simulink model "darko_control_lineaire_wind_test"  (R2021b)
settings: Solver=VariableStepAuto  StartTime=0.0  StopTime=50  RelTol=1e-3
values from neighbouring files (symbols this model uses):
  C = [C(1:7,:);C(9:12,:)]    [main_linearisation_wi.m]
  drone = generateDarko()    [equilibre.m]    (also in generateDarko.m = struct('MASS',               0.400,                      'IN; main_linearisation_wi.m)
  initial_state = [p_initial; v_initial; q_initial; omega_initial]    [main_linearisation_wi.m]
  K_complet = [K(:,1:6), zeros(4,1), K(:,7:12)]    [main_linearisation_wi.m]
  solution = fmincon(fun,x0,[],[],[],[],lb,ub, [], options)    [main_linearisation_wi.m]
  u_eq = drone.G*drone.MASS/(2*drone.Fb(1,1)) * [1;1;0;0]    [main_linearisation_wi.m]
  x_eq = [[0; 0; 0]; [0; 0; 0]; [1/sqrt(2); 0; 1/sqrt(2);0]; [0; 0; 0]]    [main_linearisation_wi.m]
  x_eq_ = [[0; 0; 0]; [0; 0; 0]; [0; 0]; [0; 0; 0]]    [main_linearisation_wi.m]
libraries: simulink_extras x11, aerolibanim x1, sharedtransform x1
settings Model: Creator=florian  LastModifiedBy=florian
settings SolverCC: AlgebraicLoopSolver=TrustRegion
settings DebuggingCC: SFMachineParentedDataDiag=warning

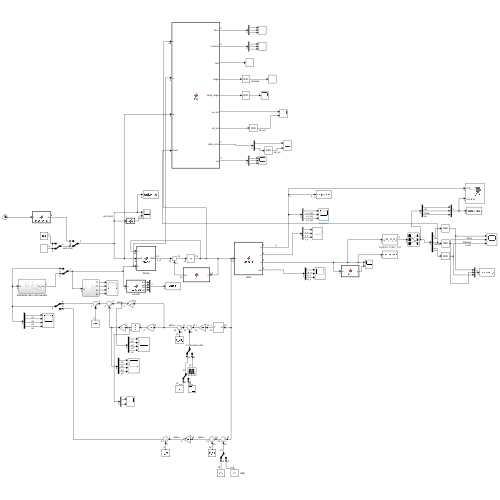
[thumbnail: Simulink's stored preview of the top-level diagram]
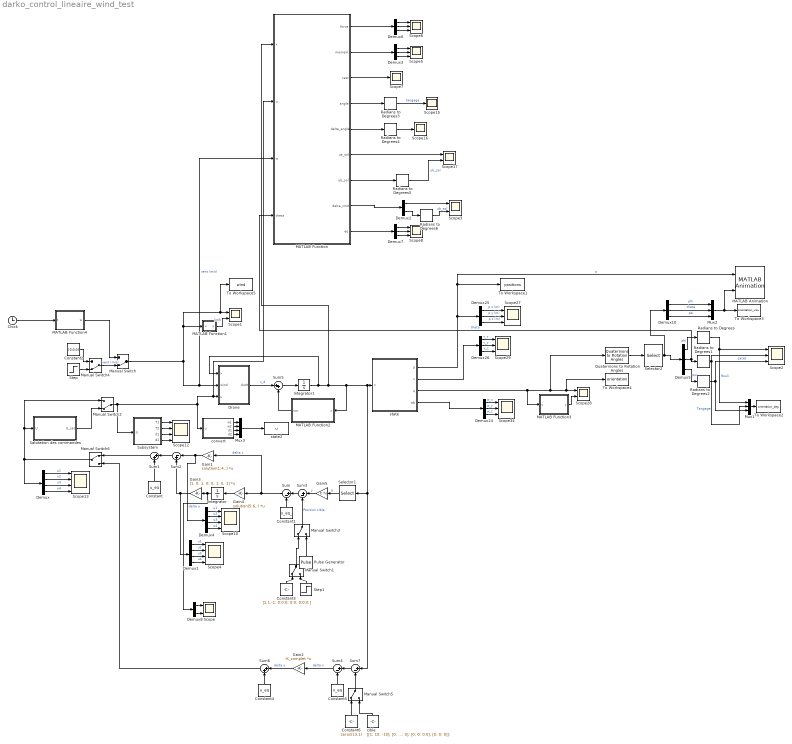
== system darko_control_lineaire_wind_test ==
  Clock : Clock
  Constant : Constant  Value=u_eq
  Constant1 : Constant  Value=x_eq_
  Constant2 : Constant  Value=[0;0;0]
  Constant3 : Constant  Value=[1;1;-1; 0;0;0; 0;0; 0;0;0;]
  Constant4 : Constant  Value=u_eq
  Constant5 : Constant  Value=x_eq
  Constant6 : Constant  Value=zeros(13,1)
  Demux : Demux
  Demux1 : Demux
  Demux{3,5..7,10,24..26} (8 alike) : Demux  Outputs=3
  Demux2 : Demux  Outputs=2
  Demux4 : Demux
  Demux8 : Demux  Outputs=2
  Drone : MATLAB Function  TreatAsAtomicUnit=on
  Gain1 : Gain  Gain=solution(1:4,:)  Multiplication=Matrix(K*u) (u vector)
  Gain2 : Gain  Gain=-K_complet  Multiplication=Matrix(K*u) (u vector)
  Gain3 : Gain  Gain=[1, 0; 1, 0; 0, 1; 0, 1]  Multiplication=Matrix(K*u) (u vector)
  Gain4 : Gain  Gain=solution(5:6,:)  Multiplication=Matrix(K*u) (u vector)
  Gain5 : Gain  Gain=C  Multiplication=Matrix(K*u) (u vector)
  Integrator : Integrator  InitialCondition=zeros(1,2)
  Integrator1 : Integrator  InitialCondition=initial_state
  MATLAB Animation : aerolibanim/MATLAB Animation  Tag=Matlab Animation 6 DOF  Vehicles=1  Geometries='astredwedge.mat'  BoundingBoxCoordinates=[-50,50,-50,50,-50,50]  CameraOffset=[0,-50,0]  CameraViewAngle=10  SampleTime=0.08  FigurePosition=[635,-23,492,413]
      settings: SourceProductBaseCode=AE
  MATLAB Function : MATLAB Function  TreatAsAtomicUnit=on
  MATLAB Function1 : MATLAB Function  TreatAsAtomicUnit=on
  MATLAB Function2 : MATLAB Function  TreatAsAtomicUnit=on
  MATLAB Function3 : MATLAB Function  TreatAsAtomicUnit=on
  MATLAB Function4 : MATLAB Function  TreatAsAtomicUnit=on
  Manual Switch : ManualSwitch  CurrentSetting=0
  Manual Switch{1,3,5..6} (4 alike) : ManualSwitch
  Manual Switch2 : ManualSwitch  CurrentSetting=0
  Manual Switch4 : ManualSwitch  CurrentSetting=0
  Mux1 : Mux  Inputs=3
  Mux2 : Mux  Inputs=3
  Mux3 : Mux
  Pulse Generator : DiscretePulseGenerator  PulseType=Time based  Amplitude=[0;0;-5; 0;0;0; 0;0; 0;0;0]  Period=5  PulseWidth=50
  Quaternions to Rotation Angles : sharedtransform/Quaternions to Rotation Angles  rotationOrder=ZXY  aMode=aMode
      settings: SourceProductBaseCode=AE,PW,DR,MT,UV,VE
  Radians to Degrees{,1..6} (7 alike) : simulink_extras/Transformations/Radians to Degrees
  Satutation des commandes : Subsystem
  Scope{,1,3,17,28} (5 alike) : Scope  NumInputPorts=2
  Scope{4,10,12..13} (4 alike) : Scope  NumInputPorts=4
  Scope15 : Scope
  Scope16 : Scope
  Scope{2,5..6,8,27,29,34} (7 alike) : Scope  NumInputPorts=3
  Scope7 : Scope
  Selector1 : Selector  InputPortWidth=13  IndexOptions=Index vector (dialog)  Indices=[1:6 8:13]  OutputSizes=1
  Selector2 : Selector  InputPortWidth=3  IndexOptions=Index vector (dialog)  Indices=[2 3 1]  OutputSizes=1
  Step : Step  Time=20  Before=[0;0;0]  After=[-4;0;0]  SampleTime=0
  Step1 : Step  Time=35  Before=zeros(11,1)  After=[-0.1;0;0; 0;0;0; 0;0; 0;0;0]  SampleTime=0
  Subsystem : Subsystem
  Sum{,3..4,7} (4 alike) : Sum  Inputs=|+-
  Sum1 : Sum  Inputs=|++
  Sum2 : Sum  Inputs=|-+
  Sum5 : Sum  Inputs=|++
  Sum6 : Sum  Inputs=|++
  To Workspace1 : ToWorkspace  VariableName=positions  SampleTime=-1
  To Workspace2 : ToWorkspace  VariableName=orientation_deg  SampleTime=-1
  To Workspace3 : ToWorkspace  VariableName=orientation_visu  SampleTime=-1
  To Workspace4 : ToWorkspace  VariableName=orientation  SampleTime=-1
  To Workspace5 : ToWorkspace  VariableName=wind  SampleTime=-1
  cible : Constant  Value=[[1; 10; -10]; [0; 0; 0]; [0; 0; 0;0]; [0; 0; 0]];
  convert : MATLAB Function  TreatAsAtomicUnit=on
  state : MATLAB Function  TreatAsAtomicUnit=on
  state2 : ToWorkspace  VariableName=u  SampleTime=-1
  wires:
  Sum5/1 -> Integrator1/1
  MATLAB Function2/1(cor) -> Sum5/2
  Drone/1(dxdt) -> Sum5/1  "x_d"
  Integrator1/1 -> Drone/1(x), MATLAB Function/1(x), Sum7/1, Selector1/1, state/1(x), MATLAB Function2/1(x)
  Demux25/3 -> Scope27/3  "p z (m)"
  Demux26/2 -> Scope29/2  "v_y"
  Demux24/1 -> Scope34/1  "w_x"
  MATLAB Function3/1(y) -> Scope28/2
  Demux25/1 -> Scope27/1  "p x (m)"
  state/4(wb) -> Demux24/1
  Demux24/2 -> Scope34/2  "w_y"
  Demux24/3 -> Scope34/3  "w_z"
  state/2(v) -> Demux26/1
  Demux25/2 -> Scope27/2  "p y (m)"
  Demux26/3 -> Scope29/3  "v_z"
  Demux26/1 -> Scope29/1  "v_x"
  Constant/1 -> Sum1/2
  Constant1/1 -> Sum/2
  Demux5/2 -> MATLAB Function/4(theta), Radians to Degrees1/1  "theta"
  Demux5/1 -> Radians to Degrees/1  "phi"
  Demux5/3 -> Radians to Degrees2/1  "psi"
  Demux/3 -> Scope13/3  "u3"
  Manual Switch6/1 -> Demux/1, Satutation des commandes/1(U), Manual Switch2/1
  Demux/2 -> Scope13/2  "u2"
  Manual Switch2/1 -> Subsystem/1(U), convert/1(u), MATLAB Function/2(u), Drone/3(u)
  Demux/1 -> Scope13/1  "u1"
  Demux/4 -> Scope13/4  "u4"
  Mux1/1 -> To Workspace2/1
  state/3(q) -> Quaternions to Rotation Angles/1, Scope28/1, To Workspace4/1, MATLAB Function3/1(u)
  Satutation des commandes/1(U_sat) -> Manual Switch2/2
  Demux10/2 -> Mux2/2  "theta"
  Selector2/1 -> Demux10/1, Demux5/1
  Demux10/1 -> Mux2/1  "phi"
  Demux10/3 -> Mux2/3  "psi"
  state/1(p) -> Demux25/1, MATLAB Animation/1, To Workspace1/1  "p"
  Mux2/1 -> To Workspace3/1, MATLAB Animation/2
  Manual Switch/1 -> MATLAB Function/3(w), Drone/2(wind), To Workspace5/1, Scope1/1, MATLAB Function1/1(u)  "vent (m/s)"
  Radians to Degrees1/1 -> Mux1/2, Scope2/2  "Tangage"
  Radians to Degrees/1 -> Scope2/1, Mux1/1  "Rouli"
  Radians to Degrees2/1 -> Scope2/3, Mux1/3  "Lacet"
  Integrator/1 -> Demux8/1, Gain3/1
  Sum/1 -> Gain4/1, Gain1/1  "delta x"
  Gain4/1 -> Integrator/1
  Sum2/1 -> Sum1/1
  Gain1/1 -> Demux4/1, Sum2/1  "delta u"
  Demux1/2 -> Scope4/2  "u2"
  Demux1/3 -> Scope4/3  "u3"
  Demux1/4 -> Scope4/4  "u4"
  Demux1/1 -> Scope4/1  "u1"
  Gain5/1 -> Sum3/1  "y"
  Sum3/1 -> Sum/1
  convert/1(w1) -> Mux3/1
  Mux3/1 -> state2/1
  convert/2(w2) -> Mux3/2
  convert/3(d1) -> Mux3/3
  convert/4(d2) -> Mux3/4
  Gain3/1 -> Sum2/2, Demux1/1
  Demux4/2 -> Scope10/2  "u2"
  Demux4/3 -> Scope10/3  "u3"
  Demux4/4 -> Scope10/4  "u4"
  Demux4/1 -> Scope10/1  "u1"
  Step/1 -> Manual Switch4/2
  Subsystem/1(T1) -> Scope12/1
  Subsystem/4(d2) -> Scope12/4
  Subsystem/2(T2) -> Scope12/2
  Subsystem/3(d1) -> Scope12/3
  Constant2/1 -> Manual Switch4/1
  Demux6/2 -> Scope6/2
  Radians to Degrees5/1 -> Scope17/2  "ub_sol"
  Demux6/3 -> Scope6/3
  Radians to Degrees4/1 -> Scope16/1
  MATLAB Function/5(delta_angle) -> Radians to Degrees4/1
  MATLAB Function/2(moment) -> Demux3/1
  MATLAB Function/8(delta_cmd) -> Demux2/1
  Radians to Degrees3/1 -> Scope15/1  "tangage"
  MATLAB Function/4(angle) -> Radians to Degrees3/1
  MATLAB Function/7(ub_sol) -> Radians to Degrees5/1
  MATLAB Function/6(ua_sol) -> Scope17/1
  Demux2/1 -> Scope3/1
  MATLAB Function/1(force) -> Demux6/1
  Radians to Degrees6/1 -> Scope3/2  "ub_sol"
  MATLAB Function/3(test) -> Scope7/1
  Demux3/3 -> Scope5/3
  Demux2/2 -> Radians to Degrees6/1
  Demux6/1 -> Scope6/1
  Demux3/1 -> Scope5/1
  Demux3/2 -> Scope5/2
  Demux7/3 -> Scope8/3
  MATLAB Function/9(eq) -> Demux7/1
  Demux7/1 -> Scope8/1
  Demux7/2 -> Scope8/2
  MATLAB Function1/1(y) -> Scope1/2  "kmh"
  Step1/1 -> Manual Switch1/2
  Constant3/1 -> Manual Switch1/1
  Pulse Generator/1 -> Manual Switch3/2
  Manual Switch1/1 -> Manual Switch3/1
  Manual Switch3/1 -> Sum3/2  "Position cible"
  Quaternions to Rotation Angles/1 -> Selector2/1
  Manual Switch4/1 -> Manual Switch/2  "vent (m/s)"
  Clock/1 -> MATLAB Function4/1(t)
  MATLAB Function4/1(w) -> Manual Switch/1
  Selector1/1 -> Gain5/1  "p"
  Sum4/1 -> Gain2/1  "delta x"
  Gain2/1 -> Sum6/1  "delta u"
  Constant4/1 -> Sum6/2
  cible/1 -> Manual Switch5/2
  Constant5/1 -> Sum4/2
  Sum7/1 -> Sum4/1
  Manual Switch5/1 -> Sum7/2
  Sum6/1 -> Manual Switch6/2
  Constant6/1 -> Manual Switch5/1
  Sum1/1 -> Manual Switch6/1
  Demux8/2 -> Scope/2
  Demux8/1 -> Scope/1

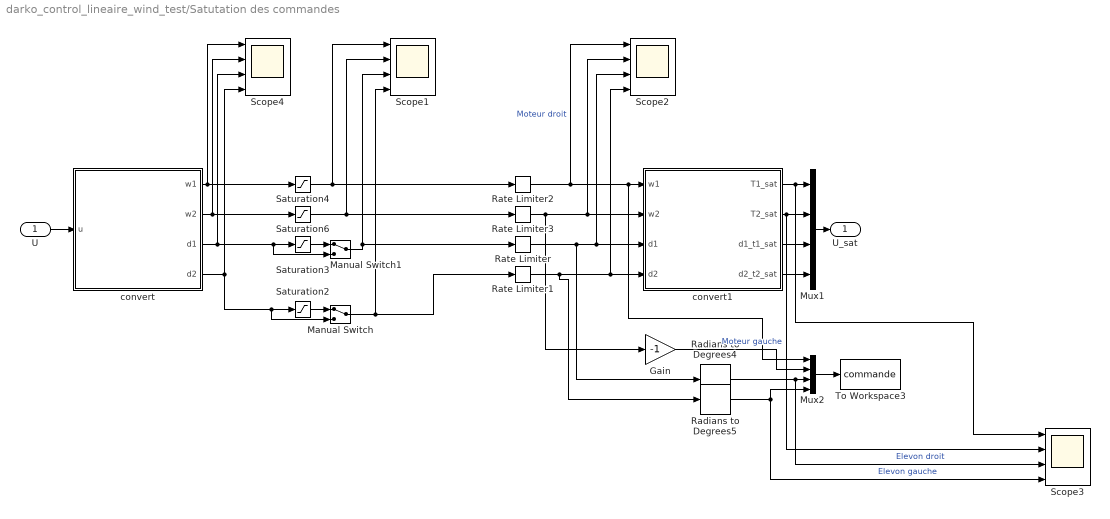
== system darko_control_lineaire_wind_test/Satutation des commandes ==
  U : Inport
  Gain : Gain  Gain=-1
  Manual Switch : ManualSwitch
  Manual Switch1 : ManualSwitch
  Mux1 : Mux
  Mux2 : Mux
  Radians to Degrees4 : simulink_extras/Transformations/Radians to Degrees
  Radians to Degrees5 : simulink_extras/Transformations/Radians to Degrees
  Rate Limiter : RateLimiter  RisingSlewLimit=drone.ELEVON_RATE_CHANGE  FallingSlewLimit=-drone.ELEVON_RATE_CHANGE  SampleTimeMode=inherited
  Rate Limiter1 : RateLimiter  RisingSlewLimit=drone.ELEVON_RATE_CHANGE  FallingSlewLimit=-drone.ELEVON_RATE_CHANGE  SampleTimeMode=inherited
  Rate Limiter2 : RateLimiter  RisingSlewLimit=drone.MOTOR_RATE_CHANGE  FallingSlewLimit=-drone.MOTOR_RATE_CHANGE  SampleTimeMode=inherited
  Rate Limiter3 : RateLimiter  RisingSlewLimit=drone.MOTOR_RATE_CHANGE  FallingSlewLimit=-drone.MOTOR_RATE_CHANGE  SampleTimeMode=inherited
  Saturation2 : Saturate  UpperLimit=30*(pi/180)  LowerLimit=-30*(pi/180)
  Saturation3 : Saturate  UpperLimit=30*(pi/180)  LowerLimit=-30*(pi/180)
  Saturation4 : Saturate  UpperLimit=2000  LowerLimit=200
  Saturation6 : Saturate  UpperLimit=2000  LowerLimit=200
  Scope{1..4} (4 alike) : Scope  NumInputPorts=4
  To Workspace3 : ToWorkspace  VariableName=commande  SampleTime=-1
  convert : MATLAB Function  TreatAsAtomicUnit=on
  convert1 : MATLAB Function  TreatAsAtomicUnit=on
  U_sat : Outport
  wires:
  convert/1(w1) -> Saturation4/1, Scope4/1
  convert/2(w2) -> Scope4/2, Saturation6/1
  convert/3(d1) -> Scope4/3, Manual Switch1/2, Saturation3/1
  convert/4(d2) -> Manual Switch/2, Saturation2/1, Scope4/4
  convert1/1(T1_sat) -> Scope3/1, Mux1/1
  convert1/4(d2_t2_sat) -> Mux1/4
  Mux1/1 -> U_sat/1
  convert1/2(T2_sat) -> Scope3/2, Mux1/2
  convert1/3(d1_t1_sat) -> Mux1/3
  Saturation6/1 -> Rate Limiter3/1, Scope1/2
  Saturation4/1 -> Rate Limiter2/1, Scope1/1
  U/1 -> convert/1(u)
  Radians to Degrees5/1 -> Mux2/4, Scope3/4  "Elevon gauche"
  Rate Limiter3/1 -> Gain/1, convert1/2(w2), Scope2/2
  Rate Limiter1/1 -> Radians to Degrees5/1, Scope2/4, convert1/4(d2)
  Rate Limiter/1 -> Radians to Degrees4/1, Scope2/3, convert1/3(d1)
  Gain/1 -> Mux2/2  "Moteur gauche"
  Mux2/1 -> To Workspace3/1
  Radians to Degrees4/1 -> Scope3/3, Mux2/3  "Elevon droit"
  Rate Limiter2/1 -> Scope2/1, Mux2/1, convert1/1(w1)  "Moteur droit"
  Saturation3/1 -> Manual Switch1/1
  Manual Switch1/1 -> Rate Limiter/1, Scope1/3
  Saturation2/1 -> Manual Switch/1
  Manual Switch/1 -> Scope1/4, Rate Limiter1/1

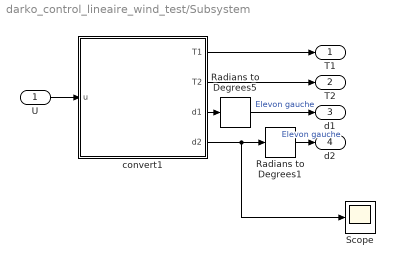
== system darko_control_lineaire_wind_test/Subsystem ==
  U : Inport
  Radians to Degrees1 : simulink_extras/Transformations/Radians to Degrees
  Radians to Degrees5 : simulink_extras/Transformations/Radians to Degrees
  Scope : Scope
  convert1 : MATLAB Function  TreatAsAtomicUnit=on
  T1 : Outport
  T2 : Outport  Port=2
  d1 : Outport  Port=3
  d2 : Outport  Port=4
  wires:
  U/1 -> convert1/1(u)
  convert1/1(T1) -> T1/1
  convert1/2(T2) -> T2/1
  Radians to Degrees5/1 -> d1/1  "Elevon gauche"
  convert1/3(d1) -> Radians to Degrees5/1
  Radians to Degrees1/1 -> d2/1  "Elevon gauche"
  convert1/4(d2) -> Scope/1, Radians to Degrees1/1

== matlab function darko_control_lineaire_wind_test/Satutation des commandes/convert1 ==
  data: w1 input; w2 input; d1 input; d2 input; T1_sat output; T2_sat output; drone parameter; d1_t1_sat output; d2_t2_sat output
function [T1_sat, T2_sat, d1_t1_sat, d2_t2_sat] = convert2(w1, w2, d1, d2, drone)
%#codegen
kf = drone.PROP_KP;

T1_sat = kf*w1^2;
d1_t1_sat = d1*T1_sat;
T2_sat = kf*w2^2;
d2_t2_sat = d2*T2_sat;

== matlab function darko_control_lineaire_wind_test/MATLAB Function2 ==
  data: x input; cor output
function cor  = fcn(x)
%#codegen
q  = x(7:10);
n = norm(q);
mismatch = 1-n;
cor = [0;0;0; 0;0;0; mismatch*q; 0;0;0];

== matlab function darko_control_lineaire_wind_test/MATLAB Function3 ==
  data: u input; y output
function y = fcn(u)
%#codegen

y = norm(u);

== matlab function darko_control_lineaire_wind_test/convert ==
  data: u input; w1 output; drone parameter; w2 output; d1 output; d2 output
function [w1, w2, d1, d2] = convert(u, drone)
%#codegen
kf = drone.PROP_KP;

T1 = max(u(1),0);
T2 = max(u(2),0);
d1_T1 = u(3);
d2_T2 = u(4);

w1 = sqrt(T1/kf)*60/(2*pi);
w2 = sqrt(T2/kf)*60/(2*pi);
d1 = d1_T1/T1 *(360/(2*pi));
d2 = d2_T2/T2*(360/(2*pi));

== matlab function darko_control_lineaire_wind_test/state ==
  data: x input; p output; v output; q output; wb output
function [p, v, q, wb] = demux(x)
%#codegen

p = x(1:3);
v = x(4:6);
q  = x(7:10);
wb = x(11:13);

== matlab function darko_control_lineaire_wind_test/MATLAB Function ==
  data: force output; moment output; test output; x input; u input; w input; theta input; drone parameter; angle output; delta_angle output; ua_sol output; ub_sol output; delta_cmd output; eq output
function [force,moment, test, angle, delta_angle, ua_sol, ub_sol, delta_cmd, eq] = fcn(x, u, w, theta, drone)
%#codegen


% p = x(1:3);
vl = x(4:6);
q  = x(7:10);
wb = x(11:13);

PHI_fv = drone.PHI(1:3,1:3);
PHI_mv = drone.PHI(4:6,1:3);
PHI_mw = drone.PHI(4:6,4:6);
phi_n  = drone.PHI_n;
rho    = drone.RHO;
Swet   = drone.WET_SURFACE;
Sdry   = drone.DRY_SURFACE;
chord  = drone.CHORD;
ws     = drone.WINGSPAN;
xi_m = drone.ELEVON_MEFFICIENCY;
xi_f = drone.ELEVON_FEFFICIENCY;
a1 = drone.P_A1_CG;
a2 = drone.P_A2_CG;
Sp = pi*drone.PROP_RADIUS^2;
dR = drone.CENTRAGE ;

% gravity
g = drone.G;
% vehicle mass
m = drone.MASS;

cd0 = PHI_fv(1,1);
cl0 = PHI_fv(3,3);

S = Swet + Sdry;

D = q2dcm(q);

B = diag([ws; chord; ws]);
vinf = D'*(vl-w);

eta = sqrt( norm(vinf)^2 + phi_n*norm(B*wb)^2 );


T1 = max(u(1),0);
T2 = max(u(2),0);
d1_T1 = u(3);
d2_T2 = u(4);

d1 = d1_T1/T1;
d2 = d2_T2/T2;

ua = T1;
ub = d1;

eq1 = 2*(1-(S/(4*Sp))*cd0)*ua - 1/2*rho*S*eta*cd0*vinf(1) + 1/2*rho*S*eta*cd0*xi_f(2)*ub*vinf(3) - m*g*sin(theta);

eq2 = -1/2*rho*S*eta*cl0*vinf(3) - 1/2*rho*S*eta*cl0*xi_f(2)*ub*vinf(1) - S/(2*Sp)*xi_f(2)*cl0*ua*ub + m*g*cos(theta);

eq3 = 1/2*rho*S*dR*cl0*eta*vinf(3) + 1/2*rho*S*dR*cl0*eta*xi_m(2)*ub*vinf(1) + S/(2*Sp)*dR*cl0*xi_m(2)*ua*ub;


Fp = -1/2 * rho * S * PHI_fv * eta * vinf ...
     + 1/4 * rho * S * PHI_fv * skew_sym(xi_f) * (d1 + d2) * eta * vinf + drone.Fb*u +D'*[0;0;m*g]-1/2 * rho * S * PHI_mv * eta * B * wb + 1/4 * rho * S * PHI_mv * skew_sym(xi_f) * (d1 + d2) * B * eta * wb;

Mp = -1/2 * rho * S * B * PHI_mv * eta * vinf  ...
     + 1/4 * rho * S * skew_sym(a1) * PHI_fv * skew_sym(xi_f)* d1 * eta * vinf ...
     + 1/4 * rho * S * skew_sym(a2) * PHI_fv * skew_sym(xi_f)* d2 * eta * vinf ...
     + 1/4 * rho * S * B * PHI_mv * skew_sym(xi_m) * (d1 + d2) * eta * vinf ...
      +drone.Mb*u + 1/4 * rho * S * B * PHI_mw * skew_sym(xi_m) * (d1 + d2) * eta * B * wb - 1/2 * rho * S *B * PHI_mw * eta * wb + 1/4 * rho * S * skew_sym(a1) * PHI_mv * skew_sym(xi_f)* d1 * eta * B * eta * wb + 1/4 * rho * S * skew_sym(a2) * PHI_mv * skew_sym(xi_f)* d2 * eta * B * eta * wb; 

temp = drone.Fb*u;
test =  2*(1-(S/(4*Sp))*cd0)*ua - temp(1);


force = [eq1;0;eq2] - Fp;
moment = [0;eq3;0] - Mp;


eta2 = norm(w);


if eta2 ~= 0
    
%     angle =  [2*atan((b_theta-sqrt(a_theta^2 + b_theta^2))/a_theta), 2*atan((b_theta+sqrt(a_theta^2 + b_theta^2))/a_theta)]; % 
    angle = -atan(w(3)/w(1) - (2*m*g)/(rho*S*cl0*eta2*((xi_f(2)/xi_m(2))-1)*w(1)));

    
    delta_angle = theta -  angle;

    w_barre  = [cos(angle), 0, -sin(angle); 0, 1, 0; sin(angle), 0, cos(angle)]*(-w);
    wx_barre = w_barre(1);
    wz_barre = w_barre(3);


%     a = 2*(1-(S*cd0)/(4*Sp));
%     b = 1/2*rho*S*eta2*cd0*xi_f(2)*wz_barre;
%     c = -1/2*rho*S*eta2*cd0*wx_barre - m*g*sin(angle);
% 
%     d =  -1/2*rho*S*eta2*cl0*xi_f(2)*wx_barre;
%     e = - S/(2*Sp)*xi_f(2)*cl0;
%     f = -1/2*rho*S*eta2*cl0*wz_barre + m*g*cos(angle);
% % 
% %     ua_sol = (-sqrt(a^2*d^2 + 4*e*a*b*f + 2*e*a*c*d + e^2*c^2) - a*d + e*c)/(2*e*a);
% %     ub_sol = (sqrt(a^2*d^2 + 4*e*a*b*f + 2*e*a*c*d + e^2*c^2) + a*d + e*c)/(2*e*b);
%     ua_sol = -(sqrt(a^2*d^2 + 4*e*a*b*f + 2*e*a*c*d + e^2*c^2) - a*d + e*c)/(2*e*a);
%     ub_sol = -(-sqrt(a^2*d^2 + 4*e*a*b*f + 2*e*a*c*d + e^2*c^2) + a*d + e*c)/(2*e*b);
%     delta_cmd = [ua;ub]- [ua_sol;ub_sol];
    a = (2*(1-(S*cd0)/(4*Sp))*cl0)/(rho*Sp*eta2*cd0*wz_barre);
    b = (2*cl0*wx_barre)/(cd0*wz_barre)*(1-(S*cd0)/(4*Sp)) - (m*g*sin(angle)*cl0)/(rho*Sp*eta2*cd0*wz_barre) - (S*wx_barre*cl0)/(2*Sp*wz_barre);
    c = m*g*cos(angle) - (1/2)*rho*S*eta2*cl0*(wz_barre + (wx_barre^2)/wz_barre) - (cl0*wx_barre*m*g*sin(angle))/(cd0*wz_barre);

    ua_sol = max(real(roots([a b c])));

    ub_sol = (2*m*g*sin(angle))/(rho*S*eta2*cd0*xi_f(2)*wz_barre) + (wx_barre)/(xi_f(2)*wz_barre) - (4*(1-(S*cd0)/(4*Sp))*ua_sol)/(rho*S*eta2*cd0*xi_f(2)*wz_barre);
    delta_cmd = [ua;ub]- [ua_sol;ub_sol];

    eq = [2*(1-(S/(4*Sp))*cd0)*ua_sol - 1/2*rho*S*eta*cd0*vinf(1) + 1/2*rho*S*eta*cd0*xi_f(2)*ub_sol*vinf(3) - m*g*sin(angle);...
          -1/2*rho*S*eta*cl0*vinf(3) - 1/2*rho*S*eta*cl0*xi_f(2)*ub_sol*vinf(1) - S/(2*Sp)*xi_f(2)*cl0*ua_sol*ub_sol + m*g*cos(angle);...
          1/2*rho*S*dR*cl0*eta*vinf(3) + 1/2*rho*S*dR*cl0*eta*xi_m(2)*ub_sol*vinf(1) + S/(2*Sp)*dR*cl0*xi_m(2)*ua_sol*ub_sol ];

else
    wx_barre = 0;
    wz_barre = 0;
    angle = 0;
    delta_angle = 0;
    ua_sol = 0;
    ub_sol = 0;
    delta_cmd = [0;0];
    eq = [0;0;0];
    
   
end

== matlab function darko_control_lineaire_wind_test/Drone ==
  data: x input; wind input; u input; dxdt output; drone parameter
function dxdt  = drone(x,wind, u, drone)

%% physical constants
% gravity
g = drone.G;
% vehicle mass
m = drone.MASS;
% vehicle inertia matrix
J = drone.INERTIA; % [3x3 real symmetric] in body axis

%% state demultiplexing
% p = x(1:3);
v = x(4:6);
q  = x(7:10);
wb = x(11:13);

Rq = q2dcm(q);

[Fp, Mp] = external_force_moment(x, u, wind, drone);

% position
dpdt = v;

% kinematics
dvdt =  [0;0;g] + (1/m)*Rq*drone.Fb*u + (1/m)*Rq*Fp; 

%% quaternion derivative
eta = q(1);
eps = q(2:4);

dqdt = (1/2)*[-eps'; eta*eye(3) + skew_sym(eps)]*wb;

%% angular velocity derivative
% kinematics
dwdt = -J\cross(wb, J*wb) + J\(drone.Mb*u) + J\Mp;


%% derivative multiplexing
dxdt = [dpdt; dvdt; dqdt; dwdt] ;

== matlab function darko_control_lineaire_wind_test/Subsystem/convert1 ==
  data: u input; T1 output; drone parameter; T2 output; d1 output; d2 output
function [T1, T2, d1, d2] = convert(u, drone)
%#codegen
kf = drone.PROP_KP;

T1 = max(u(1),0);
T2 = max(u(2),0);
d1_T1 = u(3);
d2_T2 = u(4);

w1 = sqrt(T1/kf);
w2 = sqrt(T2/kf);
d1 = d1_T1/T1;
d2 = d2_T2/T2;

== matlab function darko_control_lineaire_wind_test/MATLAB Function1 ==
  data: u input; y output
function y = nor(u)
%#codegen

y = norm(u)*3.6;

== matlab function darko_control_lineaire_wind_test/MATLAB Function4 ==
  data: t input; w output
function w = mex_wind(t)
%#codegen
t0 = 10; %s
wx_mean = 3;
fg = 0.8;
Ag = -4; %m/s
if (t-t0)<0 ||  (t-t0)> 1/fg
    wx = wx_mean;
else
    wx = wx_mean + (Ag/2)*(1-cos(2*pi*fg*(t-t0)))*sin(3*pi*fg*(t-t0));
end
w = [-wx;0;0];

== matlab function darko_control_lineaire_wind_test/Satutation des commandes/convert ==
  data: u input; w1 output; drone parameter; w2 output; d1 output; d2 output
function [w1, w2, d1, d2] = convert(u, drone)
%#codegen
kf = drone.PROP_KP;

T1 = max(u(1),0);
T2 = max(u(2),0);
d1_T1 = u(3);
d2_T2 = u(4);

w1 = sqrt(T1/kf);
w2 = sqrt(T2/kf);
d1 = d1_T1/T1;
d2 = d2_T2/T2;
